simulink model "adxl_read"  (R2024a)
settings: Solver=FixedStepAuto  StartTime=0.0  StopTime=inf  FixedStep=0.01  RelTol=1e-3  EnableMultiTasking=on
InitFcn:
  | angleEstRate = 0.01;
undefined symbols (not defined in the file or in its folder): bits
libraries: stm32blockslib x22
settings Model: STM32="{\"I2CControllerRead\":[{\"ID\":\"adxl_read:13\"},{\"ID\":\"adxl_read:12\"},{\"ID\":\"adxl_read:11\"},{\"ID\":\"adxl_read:10\"},{\"ID\":\"adxl_read:9\"},{\"ID\":\"adxl_read:8\"},{\"ID\":\"adxl_read:6\"},{\"ID\":\"adxl_read:7\"},{\"ID\":\"adxl_read:87\"},{\"ID\":\"adxl_read:84\"},{\"ID\":\"adxl_read:85\"},{\"ID\":\"adxl_read:86\"},{\"ID\":\"adxl_read:88\"},{\"ID\":\"adxl_read:89\"},{\"ID\":\"adxl_read:63\"},{\"ID\":\"adxl_read:64\"},{\"ID\":\"adxl_read:65\"}],\"I2CControllerWrite\":[{\"ID\":\"adxl_read:14\"},{\"ID\":\"adxl_read:15\"},{\"ID\":\"adxl_read:66\"},{\"ID\":\"adxl_read:67\"},{\"ID\":\"adxl_read:68\"}]}"  Creator=Peter  LastModifiedBy=Peter
settings OptimizationCC: EnhancedBackFolding=on  PassReuseOutputArgsAs=Individual arguments  ZeroExternalMemoryAtStartup=off  ZeroInternalMemoryAtStartup=off  MaxStackSize=64  OptimizeBlockOrder=speed  DifferentSizesBufferReuse=on  OptimizationCustomize=off  EfficientTunableParamExpr=on
settings DebuggingCC: ParameterTunabilityLossMsg=error
settings HardwareCC: ProdBitPerPointer=32  ProdBitPerSizeT=32  ProdBitPerPtrDiffT=32  ProdLargestAtomicInteger=Long  ProdLargestAtomicFloat=Double  ProdWordSize=32  ProdLongLongMode=on  ProdHWDeviceType=ARM Compatible->ARM Cortex-M
settings SFSimCC: MATLABDynamicMemAlloc=off
settings RTWCC: Description=Embedded Coder  SystemTargetFile=ert.tlc  HardwareBoard=STM32F7xx Based (Single precision FPU)  GenCodeOnly=on  TemplateMakefile=ert_default_tmf  Toolchain=GNU Tools for ARM Embedded Processors
settings CodeAppCC: ForceParamTrailComments=on  IgnoreCustomStorageClasses=off  OperatorAnnotations=on  SimulinkDataObjDesc=on  SFDataObjDesc=on  InsertBlockDesc=on
settings ERTTargetCC: TargetLangStandard=C99 (ISO)  CodeReplacementLibrary=ARM Cortex-M  ExtModeTransport=3  ExtModeStaticAlloc=on  ExtModeStaticAllocSize=2048  ExtModeMexFile=ext_xcp  ExtModeIntrfLevel=Level2 - Open

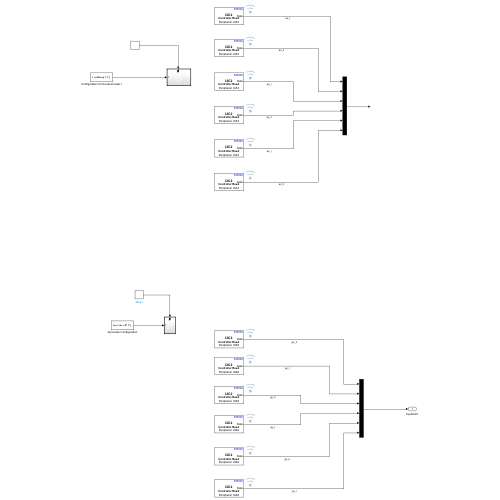
[thumbnail: Simulink's stored preview of the top-level diagram]
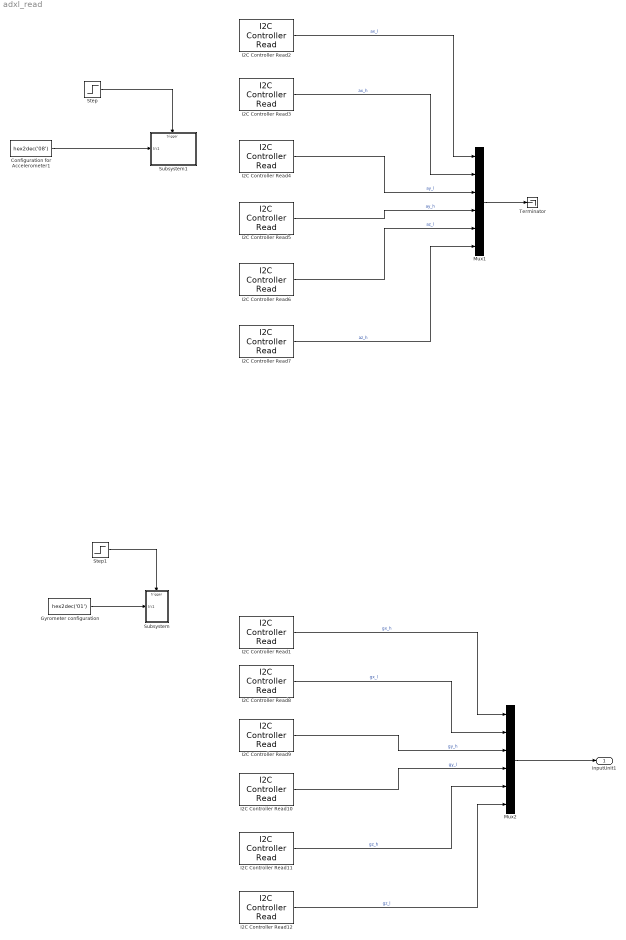
== system adxl_read ==
  Configuration for Accelerometer1 : Constant  Value=hex2dec('08')  OutDataTypeStr=uint8
  Gyrometer configuration : Constant  Value=hex2dec('01')  OutDataTypeStr=uint8
  I2C Controller Read1 : stm32blockslib/I2C Controller Read  I2CModule=I2C2  Mode=Controller  AddressingMode=7-bits  PeripheralByteOrder=LittleEndian  OwnPeripheralAddress=uint8(170)  PeripheralAddressVia=Dialog  PeripheralAddress=hex2dec('68')  RegisterAddressMode=on  RegisterAddressVia=Dialog  RegisterAddress=uint8(hex2dec('1D'))  RepeatedStart=off  NoAck=off  OutputStatus=off  BlockMode=Receive  DataType=uint8  DataLength=1  Timeout=0.001  SampleTime=angleEstRate
      settings: LibrarySourceBlock=stm32f7xxblockslib/I2C Controller Read
  I2C Controller Read10 : stm32blockslib/I2C Controller Read  I2CModule=I2C2  Mode=Controller  AddressingMode=7-bits  PeripheralByteOrder=LittleEndian  OwnPeripheralAddress=uint8(170)  PeripheralAddressVia=Dialog  PeripheralAddress=hex2dec('68')  RegisterAddressMode=on  RegisterAddressVia=Dialog  RegisterAddress=uint8(hex2dec('20'))  RepeatedStart=off  NoAck=off  OutputStatus=off  BlockMode=Receive  DataType=uint8  DataLength=1  Timeout=0.001  SampleTime=angleEstRate
      settings: LibrarySourceBlock=stm32f7xxblockslib/I2C Controller Read
  I2C Controller Read11 : stm32blockslib/I2C Controller Read  I2CModule=I2C2  Mode=Controller  AddressingMode=7-bits  PeripheralByteOrder=LittleEndian  OwnPeripheralAddress=uint8(170)  PeripheralAddressVia=Dialog  PeripheralAddress=hex2dec('68')  RegisterAddressMode=on  RegisterAddressVia=Dialog  RegisterAddress=uint8(hex2dec('21'))  RepeatedStart=off  NoAck=off  OutputStatus=off  BlockMode=Receive  DataType=uint8  DataLength=1  Timeout=0.001  SampleTime=angleEstRate
      settings: LibrarySourceBlock=stm32f7xxblockslib/I2C Controller Read
  I2C Controller Read12 : stm32blockslib/I2C Controller Read  I2CModule=I2C2  Mode=Controller  AddressingMode=7-bits  PeripheralByteOrder=LittleEndian  OwnPeripheralAddress=uint8(170)  PeripheralAddressVia=Dialog  PeripheralAddress=hex2dec('68')  RegisterAddressMode=on  RegisterAddressVia=Dialog  RegisterAddress=uint8(hex2dec('22'))  RepeatedStart=off  NoAck=off  OutputStatus=off  BlockMode=Receive  DataType=uint8  DataLength=1  Timeout=0.001  SampleTime=angleEstRate
      settings: LibrarySourceBlock=stm32f7xxblockslib/I2C Controller Read
  I2C Controller Read2 : stm32blockslib/I2C Controller Read  I2CModule=I2C2  Mode=Controller  AddressingMode=7-bits  PeripheralByteOrder=LittleEndian  OwnPeripheralAddress=uint8(170)  PeripheralAddressVia=Dialog  PeripheralAddress=hex2dec('53')  RegisterAddressMode=on  RegisterAddressVia=Dialog  RegisterAddress=uint8(hex2dec('32'))  RepeatedStart=off  NoAck=off  OutputStatus=off  BlockMode=Receive  DataType=uint8  DataLength=1  Timeout=0.001  SampleTime=angleEstRate
      settings: LibrarySourceBlock=stm32f7xxblockslib/I2C Controller Read
  I2C Controller Read3 : stm32blockslib/I2C Controller Read  I2CModule=I2C2  Mode=Controller  AddressingMode=7-bits  PeripheralByteOrder=LittleEndian  OwnPeripheralAddress=uint8(170)  PeripheralAddressVia=Dialog  PeripheralAddress=hex2dec('53')  RegisterAddressMode=on  RegisterAddressVia=Dialog  RegisterAddress=uint8(hex2dec('33'))  RepeatedStart=off  NoAck=off  OutputStatus=off  BlockMode=Receive  DataType=uint8  DataLength=1  Timeout=0.001  SampleTime=angleEstRate
      settings: LibrarySourceBlock=stm32f7xxblockslib/I2C Controller Read
  I2C Controller Read4 : stm32blockslib/I2C Controller Read  I2CModule=I2C2  Mode=Controller  AddressingMode=7-bits  PeripheralByteOrder=LittleEndian  OwnPeripheralAddress=uint8(170)  PeripheralAddressVia=Dialog  PeripheralAddress=hex2dec('53')  RegisterAddressMode=on  RegisterAddressVia=Dialog  RegisterAddress=uint8(hex2dec('34'))  RepeatedStart=off  NoAck=off  OutputStatus=off  BlockMode=Receive  DataType=uint8  DataLength=1  Timeout=0.001  SampleTime=angleEstRate
      settings: LibrarySourceBlock=stm32f7xxblockslib/I2C Controller Read
  I2C Controller Read5 : stm32blockslib/I2C Controller Read  I2CModule=I2C2  Mode=Controller  AddressingMode=7-bits  PeripheralByteOrder=LittleEndian  OwnPeripheralAddress=uint8(170)  PeripheralAddressVia=Dialog  PeripheralAddress=hex2dec('53')  RegisterAddressMode=on  RegisterAddressVia=Dialog  RegisterAddress=uint8(hex2dec('35'))  RepeatedStart=off  NoAck=off  OutputStatus=off  BlockMode=Receive  DataType=uint8  DataLength=1  Timeout=0.001  SampleTime=angleEstRate
      settings: LibrarySourceBlock=stm32f7xxblockslib/I2C Controller Read
  I2C Controller Read6 : stm32blockslib/I2C Controller Read  I2CModule=I2C2  Mode=Controller  AddressingMode=7-bits  PeripheralByteOrder=LittleEndian  OwnPeripheralAddress=uint8(170)  PeripheralAddressVia=Dialog  PeripheralAddress=hex2dec('53')  RegisterAddressMode=on  RegisterAddressVia=Dialog  RegisterAddress=uint8(hex2dec('36'))  RepeatedStart=off  NoAck=off  OutputStatus=off  BlockMode=Receive  DataType=uint8  DataLength=1  Timeout=0.001  SampleTime=angleEstRate
      settings: LibrarySourceBlock=stm32f7xxblockslib/I2C Controller Read
  I2C Controller Read7 : stm32blockslib/I2C Controller Read  I2CModule=I2C2  Mode=Controller  AddressingMode=7-bits  PeripheralByteOrder=LittleEndian  OwnPeripheralAddress=uint8(170)  PeripheralAddressVia=Dialog  PeripheralAddress=hex2dec('53')  RegisterAddressMode=on  RegisterAddressVia=Dialog  RegisterAddress=uint8(hex2dec('37'))  RepeatedStart=off  NoAck=off  OutputStatus=off  BlockMode=Receive  DataType=uint8  DataLength=1  Timeout=0.001  SampleTime=angleEstRate
      settings: LibrarySourceBlock=stm32f7xxblockslib/I2C Controller Read
  I2C Controller Read8 : stm32blockslib/I2C Controller Read  I2CModule=I2C2  Mode=Controller  AddressingMode=7-bits  PeripheralByteOrder=LittleEndian  OwnPeripheralAddress=uint8(170)  PeripheralAddressVia=Dialog  PeripheralAddress=hex2dec('68')  RegisterAddressMode=on  RegisterAddressVia=Dialog  RegisterAddress=uint8(hex2dec('1E'))  RepeatedStart=off  NoAck=off  OutputStatus=off  BlockMode=Receive  DataType=uint8  DataLength=1  Timeout=0.001  SampleTime=angleEstRate
      settings: LibrarySourceBlock=stm32f7xxblockslib/I2C Controller Read
  I2C Controller Read9 : stm32blockslib/I2C Controller Read  I2CModule=I2C2  Mode=Controller  AddressingMode=7-bits  PeripheralByteOrder=LittleEndian  OwnPeripheralAddress=uint8(170)  PeripheralAddressVia=Dialog  PeripheralAddress=hex2dec('68')  RegisterAddressMode=on  RegisterAddressVia=Dialog  RegisterAddress=uint8(hex2dec('1F'))  RepeatedStart=off  NoAck=off  OutputStatus=off  BlockMode=Receive  DataType=uint8  DataLength=1  Timeout=0.001  SampleTime=angleEstRate
      settings: LibrarySourceBlock=stm32f7xxblockslib/I2C Controller Read
  Mux1 : Mux  Inputs=6
  Mux2 : Mux  Inputs=6
  Step : Step  SampleTime=0.01
  Step1 : Step  SampleTime=0.01
  Subsystem : Subsystem  RTWFcnName=ITG_Init
      settings: RTWFcnNameOpts=User specified
  Subsystem1 : Subsystem  RTWFcnName=ADXL_Init
      settings: RTWFcnNameOpts=User specified
  Terminator : Terminator
  inputUnit1 : Outport  VectorParamsAs1DForOutWhenUnconnected=off
  wires:
  I2C Controller Read7/1 -> Mux1/6  "az_h"
  I2C Controller Read5/1 -> Mux1/4  "ay_h"
  I2C Controller Read6/1 -> Mux1/5  "az_l"
  I2C Controller Read4/1 -> Mux1/3  "ay_l"
  I2C Controller Read2/1 -> Mux1/1  "ax_l"
  Mux1/1 -> Terminator/1
  I2C Controller Read3/1 -> Mux1/2  "ax_h"
  Configuration for Accelerometer1/1 -> Subsystem1/1(In1)
  Step/1 -> Subsystem1/Trigger
  Mux2/1 -> inputUnit1/1
  I2C Controller Read1/1 -> Mux2/1  "gx_h"
  I2C Controller Read12/1 -> Mux2/6  "gz_l"
  I2C Controller Read9/1 -> Mux2/3  "gy_h"
  I2C Controller Read11/1 -> Mux2/5  "gz_h"
  I2C Controller Read10/1 -> Mux2/4  "gy_l"
  I2C Controller Read8/1 -> Mux2/2  "gx_l"
  Gyrometer configuration/1 -> Subsystem/1(In1)
  Step1/1 -> Subsystem/Trigger

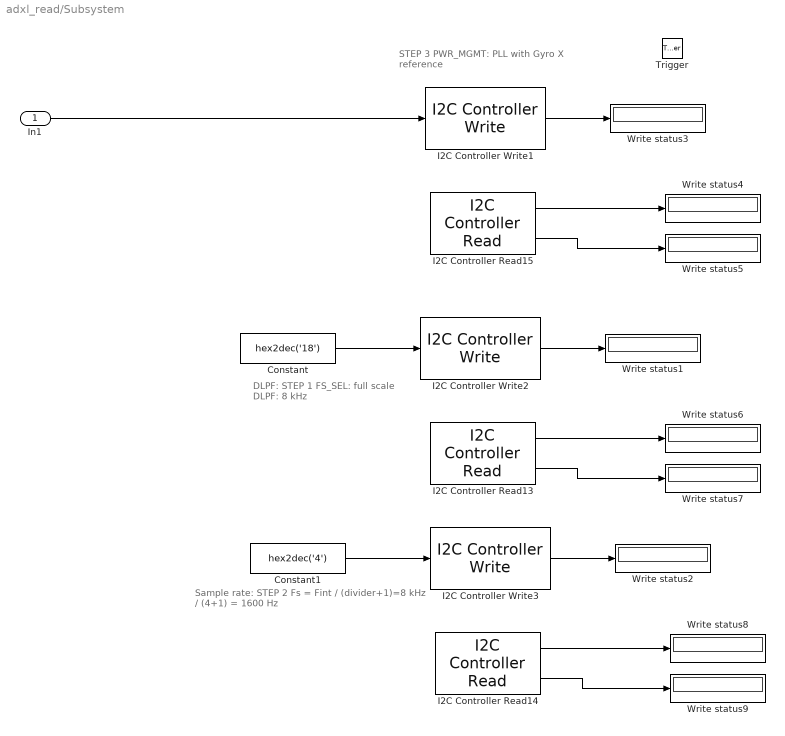
== system adxl_read/Subsystem ==
  note: STEP 3
      | PWR_MGMT: PLL with Gyro X reference
  note: Sample rate: STEP 2
      | Fs = Fint / (divider+1)=8 kHz / (4+1) = 1600 Hz
  note: DLPF: STEP 1
      | FS_SEL: full scale
      | DLPF: 8 kHz
  In1 : Inport
  Trigger : TriggerPort  VariantControl=(inherit)  PortDimensions=1
  Constant : Constant  Value=hex2dec('18')
  Constant1 : Constant  Value=hex2dec('4')
  I2C Controller Read13 : stm32blockslib/I2C Controller Read  Priority=-5  I2CModule=I2C2  Mode=Controller  AddressingMode=7-bits  PeripheralByteOrder=LittleEndian  OwnPeripheralAddress=uint8(170)  PeripheralAddressVia=Dialog  PeripheralAddress=hex2dec('68')  RegisterAddressMode=on  RegisterAddressVia=Dialog  RegisterAddress=uint8(hex2dec('16'))  RepeatedStart=off  NoAck=off  OutputStatus=on  BlockMode=Receive  DataType=uint8  DataLength=1  Timeout=0.001  SampleTime=inf
      settings: LibrarySourceBlock=stm32f7xxblockslib/I2C Controller Read
  I2C Controller Read14 : stm32blockslib/I2C Controller Read  Priority=-3  I2CModule=I2C2  Mode=Controller  AddressingMode=7-bits  PeripheralByteOrder=LittleEndian  OwnPeripheralAddress=uint8(170)  PeripheralAddressVia=Dialog  PeripheralAddress=hex2dec('68')  RegisterAddressMode=on  RegisterAddressVia=Dialog  RegisterAddress=uint8(hex2dec('15'))  RepeatedStart=off  NoAck=off  OutputStatus=on  BlockMode=Receive  DataType=uint8  DataLength=1  Timeout=0.001  SampleTime=inf
      settings: LibrarySourceBlock=stm32f7xxblockslib/I2C Controller Read
  I2C Controller Read15 : stm32blockslib/I2C Controller Read  Priority=-1  I2CModule=I2C2  Mode=Controller  AddressingMode=7-bits  PeripheralByteOrder=LittleEndian  OwnPeripheralAddress=uint8(170)  PeripheralAddressVia=Dialog  PeripheralAddress=hex2dec('68')  RegisterAddressMode=on  RegisterAddressVia=Dialog  RegisterAddress=uint8(hex2dec('3E'))  RepeatedStart=off  NoAck=off  OutputStatus=on  BlockMode=Receive  DataType=uint8  DataLength=1  Timeout=0.001  SampleTime=inf
      settings: LibrarySourceBlock=stm32f7xxblockslib/I2C Controller Read
  I2C Controller Write1 : stm32blockslib/I2C Controller Write  Priority=-2  I2CModule=I2C2  Mode=Controller  AddressingMode=7-bits  PeripheralByteOrder=LittleEndian  OwnPeripheralAddress=uint8(170)  PeripheralAddressVia=Dialog  PeripheralAddress=hex2dec('68')  RegisterAddressMode=on  RegisterAddressVia=Dialog  RegisterAddress=uint8(hex2dec('3E'))  RepeatedStart=off  NoAck=off  OutputStatus=on  BlockMode=Transmit  DataType=uint8  DataLength=1  Timeout=0.001  SampleTime=-1
      settings: LibrarySourceBlock=stm32f7xxblockslib/I2C Controller Write
  I2C Controller Write2 : stm32blockslib/I2C Controller Write  Priority=-6  I2CModule=I2C2  Mode=Controller  AddressingMode=7-bits  PeripheralByteOrder=LittleEndian  OwnPeripheralAddress=uint8(170)  PeripheralAddressVia=Dialog  PeripheralAddress=hex2dec('68')  RegisterAddressMode=on  RegisterAddressVia=Dialog  RegisterAddress=uint8(hex2dec('16'))  RepeatedStart=off  NoAck=off  OutputStatus=on  BlockMode=Transmit  DataType=uint8  DataLength=1  Timeout=0.001  SampleTime=-1
      settings: LibrarySourceBlock=stm32f7xxblockslib/I2C Controller Write
  I2C Controller Write3 : stm32blockslib/I2C Controller Write  Priority=-4  I2CModule=I2C2  Mode=Controller  AddressingMode=7-bits  PeripheralByteOrder=LittleEndian  OwnPeripheralAddress=uint8(170)  PeripheralAddressVia=Dialog  PeripheralAddress=hex2dec('68')  RegisterAddressMode=on  RegisterAddressVia=Dialog  RegisterAddress=uint8(hex2dec('15'))  RepeatedStart=off  NoAck=off  OutputStatus=on  BlockMode=Transmit  DataType=uint8  DataLength=1  Timeout=0.001  SampleTime=-1
      settings: LibrarySourceBlock=stm32f7xxblockslib/I2C Controller Write
  Write status{1..9} (9 alike) : Display
      settings: Format=hex (Stored Integer)
  wires:
  I2C Controller Write1/1 -> Write status3/1
  I2C Controller Read14/1 -> Write status8/1
  I2C Controller Read13/1 -> Write status6/1
  I2C Controller Write2/1 -> Write status1/1
  I2C Controller Read13/2 -> Write status7/1
  Constant/1 -> I2C Controller Write2/1
  In1/1 -> I2C Controller Write1/1
  I2C Controller Read14/2 -> Write status9/1
  I2C Controller Read15/1 -> Write status4/1
  I2C Controller Read15/2 -> Write status5/1
  Constant1/1 -> I2C Controller Write3/1
  I2C Controller Write3/1 -> Write status2/1

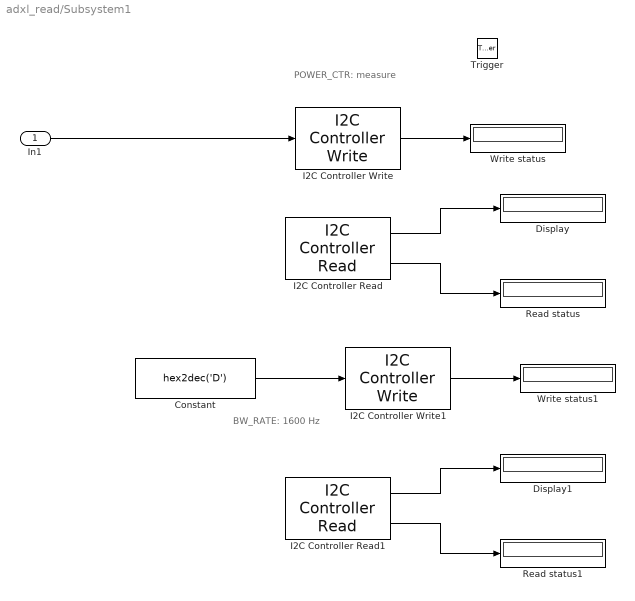
== system adxl_read/Subsystem1 ==
  note: POWER_CTR: measure
  note: BW_RATE: 1600 Hz
  In1 : Inport
  Trigger : TriggerPort  VariantControl=(inherit)  PortDimensions=1
  Constant : Constant  Value=hex2dec('D')  OutDataTypeStr=uint8
  Display : Display
      settings: Format=hex (Stored Integer)
  Display1 : Display
      settings: Format=hex (Stored Integer)
  I2C Controller Read : stm32blockslib/I2C Controller Read  Priority=-2  I2CModule=I2C2  Mode=Controller  AddressingMode=7-bits  PeripheralByteOrder=BigEndian  OwnPeripheralAddress=uint8(170)  PeripheralAddressVia=Dialog  PeripheralAddress=hex2dec('53')  RegisterAddressMode=on  RegisterAddressVia=Dialog  RegisterAddress=uint8(hex2dec('2D'))  RepeatedStart=off  NoAck=off  OutputStatus=on  BlockMode=Receive  DataType=uint8  DataLength=1  Timeout=0.001  SampleTime=inf
      settings: LibrarySourceBlock=stm32f7xxblockslib/I2C Controller Read
  I2C Controller Read1 : stm32blockslib/I2C Controller Read  Priority=-4  I2CModule=I2C2  Mode=Controller  AddressingMode=7-bits  PeripheralByteOrder=BigEndian  OwnPeripheralAddress=uint8(170)  PeripheralAddressVia=Dialog  PeripheralAddress=hex2dec('53')  RegisterAddressMode=on  RegisterAddressVia=Dialog  RegisterAddress=uint8(hex2dec('2C'))  RepeatedStart=off  NoAck=off  OutputStatus=on  BlockMode=Receive  DataType=uint8  DataLength=1  Timeout=0.001  SampleTime=inf
      settings: LibrarySourceBlock=stm32f7xxblockslib/I2C Controller Read
  I2C Controller Write : stm32blockslib/I2C Controller Write  Priority=-3  I2CModule=I2C2  Mode=Controller  AddressingMode=7-bits  PeripheralByteOrder=BigEndian  OwnPeripheralAddress=uint8(170)  PeripheralAddressVia=Dialog  PeripheralAddress=hex2dec('53')  RegisterAddressMode=on  RegisterAddressVia=Dialog  RegisterAddress=uint8(hex2dec('2D'))  RepeatedStart=off  NoAck=off  OutputStatus=on  BlockMode=Transmit  DataType=uint8  DataLength=1  Timeout=0.001  SampleTime=-1
      settings: LibrarySourceBlock=stm32f7xxblockslib/I2C Controller Write
  I2C Controller Write1 : stm32blockslib/I2C Controller Write  Priority=-5  I2CModule=I2C2  Mode=Controller  AddressingMode=7-bits  PeripheralByteOrder=BigEndian  OwnPeripheralAddress=uint8(170)  PeripheralAddressVia=Dialog  PeripheralAddress=hex2dec('53')  RegisterAddressMode=on  RegisterAddressVia=Dialog  RegisterAddress=uint8(hex2dec('2C'))  RepeatedStart=off  NoAck=off  OutputStatus=on  BlockMode=Transmit  DataType=uint8  DataLength=1  Timeout=0.001  SampleTime=-1
      settings: LibrarySourceBlock=stm32f7xxblockslib/I2C Controller Write
  Read status : Display
      settings: Format=hex (Stored Integer)
  Read status1 : Display
      settings: Format=hex (Stored Integer)
  Write status : Display
      settings: Format=hex (Stored Integer)
  Write status1 : Display
      settings: Format=hex (Stored Integer)
  wires:
  I2C Controller Write1/1 -> Write status1/1
  I2C Controller Read/1 -> Display/1
  I2C Controller Read1/2 -> Read status1/1
  In1/1 -> I2C Controller Write/1
  I2C Controller Write/1 -> Write status/1
  Constant/1 -> I2C Controller Write1/1
  I2C Controller Read/2 -> Read status/1
  I2C Controller Read1/1 -> Display1/1
